simulink model "position_control"  (R2025b)
settings: Solver=VariableStepAuto  StartTime=0.0  StopTime=Stop_Time  MaxStep=1e-3  RelTol=1e-3
values from neighbouring files (symbols this model uses):
  Battery_Voltage = 7.0    (= 7)    [motor_params.m]
  Disturbance_Time = 3.0    (= 3)    [motor_params.m]
  Disturbance_V = 0    [motor_params.m]
  K = K1    (= 2.2)    [motor_params.m]
  Ki_pos = 2.0    (= 2)    [motor_params.m]
  Kp_pos = 5.0    (= 5)    [motor_params.m]
  Kp_vel = 3.2    [motor_params.m]
  MAX_SPEED = 6.0    (= 6)    [motor_params.m]
  sigma = sigma1    (= 5)    [motor_params.m]
libraries: slpidlib x1
settings Model: Creator=henry  LastModifiedBy=henry

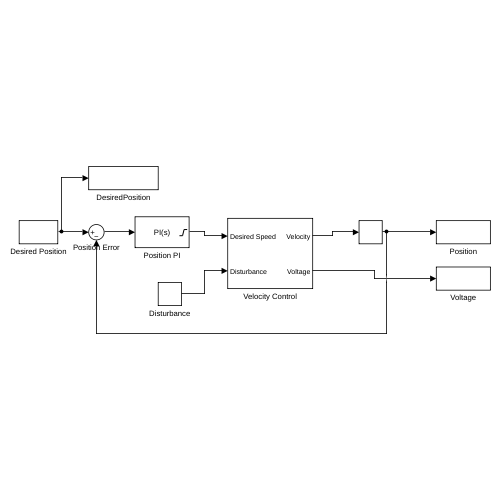
[thumbnail: Simulink's stored preview of the top-level diagram]
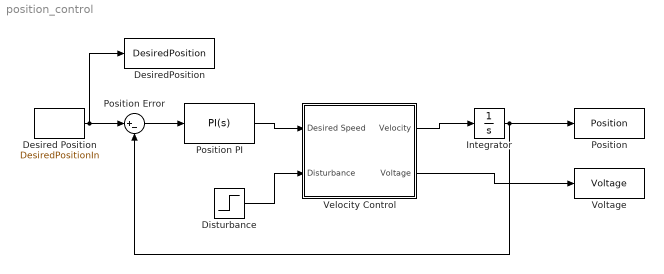
== system position_control ==
  Desired Position : FromWorkspace  VariableName=DesiredPositionIn  Interpolate=off  OutputAfterFinalValue=Holding final value
  DesiredPosition : ToWorkspace  VariableName=DesiredPosition  SaveFormat=Timeseries  SampleTime=-1
  Disturbance : Step  Time=Disturbance_Time  After=Disturbance_V  SampleTime=0
  Integrator : Integrator
  Position : ToWorkspace  VariableName=Position  SaveFormat=Timeseries  SampleTime=-1
  Position Error : Sum  Inputs=|+-
  Position PI : slpidlib/PID Controller  Controller=PI  Form=Parallel  TimeDomain=Continuous-time  UseExternalTs=off  SampleTime=-1  IntegratorMethod=Forward Euler  FilterMethod=Forward Euler  ControllerParametersSource=internal  P=Kp_pos  I=Ki_pos  UseKiTs=off  D=0  UseExternalDerivativeSource=off  N=100  UseFilter=on  TunerSelectOption=Transfer Function Based (PID Tuner App)  InitialConditionSource=internal  InitialConditionForIntegrator=0  InitialConditionForFilter=0  DifferentiatorICPrevScaledInput=0  ExternalReset=none  TrackingMode=off  Kt=1  LimitOutput=on  SatLimitsSource=internal  UpperSaturationLimit=MAX_SPEED  LowerSaturationLimit=-MAX_SPEED  LinearizeAsGain=on  AntiWindupMode=clamping  Kb=1  LimitIntegrator=off  UpperIntegratorSaturationLimit=inf  LowerIntegratorSaturationLimit=-inf  POutMin=[]  POutMax=[]  IOutMin=[]  IOutMax=[]  DOutMin=[]  DOutMax=[]  NOutMin=[]  NOutMax=[]  SumOutMin=[]  SumOutMax=[]  SaturationOutMin=[]  SaturationOutMax=[]  PParamMin=[]  PParamMax=[]  IParamMin=[]  IParamMax=[]  DParamMin=[]  DParamMax=[]  NParamMin=[]  NParamMax=[]  KbParamMin=[]  KbParamMax=[]  KtParamMin=[]  KtParamMax=[]  KbOutMin=[]  KbOutMax=[]  KtOutMin=[]  KtOutMax=[]  IntegratorOutMin=[]  IntegratorOutMax=[]  FilterOutMin=[]  FilterOutMax=[]  SumI1OutMin=[]  SumI1OutMax=[]  SumI2OutMin=[]  SumI2OutMax=[]  SumI3OutMin=[]  SumI3OutMax=[]  SumI4OutMin=[]  SumI4OutMax=[]  SumDOutMin=[]  SumDOutMax=[]  DifferentiatorOutMin=[]  DifferentiatorOutMax=[]  FilterDiffOutCoefMin=[]  FilterDiffOutCoefMax=[]  ReciprocalOutMin=[]  ReciprocalOutMax=[]  SumDenOutMin=[]  SumDenOutMax=[]  SumNumOutMin=[]  SumNumOutMax=[]  DivideOutMin=[]  DivideOutMax=[]  UdiffTsProdOutMin=[]  UdiffTsProdOutMax=[]  NTsProdOutMin=[]  NTsProdOutMax=[]  UintegralTsProdOutMin=[]  UintegralTsProdOutMax=[]  UngainTsProdOutMin=[]  UngainTsProdOutMax=[]  ClampingZeroOutDataTypeStr=Inherit: Inherit via back propagation  ClampingZeroOutMin=[]  ClampingZeroOutMax=[]  FilterDenConstantOutDataTypeStr=Inherit: Inherit via back propagation  FilterDenConstantOutMin=[]  FilterDenConstantOutMax=[]  PCopyOutDataTypeStr=Inherit: Inherit via back propagation  PCopyOutMin=[]  PCopyOutMax=[]  NCopyOutDataTypeStr=Inherit: Inherit via back propagation  NCopyOutMin=[]  NCopyOutMax=[]  IntegratorContinuousStateAttributes=''  IntegratorStateMustResolveToSignalObject=off  IntegratorRTWStateStorageClass=Auto  FilterContinuousStateAttributes=''  FilterStateMustResolveToSignalObject=off  FilterRTWStateStorageClass=Auto  ParallelPVariant=InternalParameters  IdealPVariant=Disabled  IVariant=InternalParameters  DVariant=Disabled  IntegratorVariant=Continuous  SatVariant=Enabled  AWVariant=ContClampingParallel  PCopyVariant=Disabled  TRVariant=Disabled  FdbkBlocksVariant=Forward  IdealPFdbkVariant=Disabled  SatFdbkVariant=Disabled  DerivativeFilterVariant=Disabled  NVariant=Disabled  NCopyVariant=Disabled_SignalSpec  FilterICVariant=Disabled  IntegratorICVariant=InternalICs  ExternalResetVariant=Disabled  TRSumVariant=Passthrough  SumFdbkVariant=Disabled  SumVariant=Sum_PI  TsampFilterVariant=InternalTs  TsampNgainVariant=Passthrough  TsampIntegralVariant=Disabled_SignalSpec  ExternalSaturationOutDataTypeStr=Inherit: Same as second input  DerivativeSourceVariant=Disabled  PreIntVariant=InternalPreInt
  Velocity Control : Subsystem
  Voltage : ToWorkspace  VariableName=Voltage  SaveFormat=Timeseries  SampleTime=-1
  wires:
  Desired Position/1 -> Position Error/1, DesiredPosition/1
  Position Error/1 -> Position PI/1
  Position PI/1 -> Velocity Control/1(Desired Speed)
  Disturbance/1 -> Velocity Control/2(Disturbance)
  Velocity Control/1(Velocity) -> Integrator/1
  Velocity Control/2(Voltage) -> Voltage/1
  Integrator/1 -> Position/1, Position Error/2

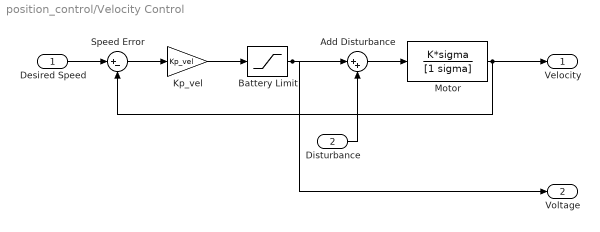
== system position_control/Velocity Control ==
  Desired Speed : Inport
  Disturbance : Inport  Port=2
  Add Disturbance : Sum  Inputs=|++
  Battery Limit : Saturate  UpperLimit=Battery_Voltage  LowerLimit=-Battery_Voltage
  Kp_vel : Gain  Gain=Kp_vel
  Motor : TransferFcn  Numerator=K*sigma  Denominator=[1 sigma]
  Speed Error : Sum  Inputs=|+-
  Velocity : Outport
  Voltage : Outport  Port=2
  wires:
  Desired Speed/1 -> Speed Error/1
  Speed Error/1 -> Kp_vel/1
  Kp_vel/1 -> Battery Limit/1
  Battery Limit/1 -> Add Disturbance/1, Voltage/1
  Disturbance/1 -> Add Disturbance/2
  Add Disturbance/1 -> Motor/1
  Motor/1 -> Velocity/1, Speed Error/2
